simulink model "rwa_power_model_test"  (R2018b)
settings: Solver=VariableStepAuto  StartTime=0.0  StopTime=10.0  RelTol=1e-3
undefined symbols (not defined in the file): simParams
libraries: rwa_power_lib x1, rwa_zero_torque_power_lib x1
settings Model: Creator=Taylor  LastModifiedBy=Taylor

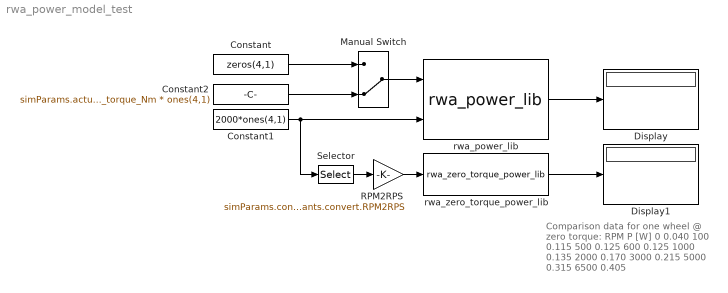
== system rwa_power_model_test ==
  note: Comparison data for one wheel
      | @ zero torque:
      |
      | RPM
      | P [W]
      |
      | 0
      | 0.040
      |
      | 100
      | 0.115
      |
      | 500
      | 0.125
      |
      | 600
      | 0.125
      |
      | 1000
      | 0.135
      |
      | 2000
      | 0.170
      |
      | 3000
      | 0.215
      |
      | 5000
      | 0.315
      |
      | 6500
      | 0.405
  Constant : Constant  Value=zeros(4,1)
  Constant1 : Constant  Value=2000*ones(4,1)
  Constant2 : Constant  Value=simParams.actuators.rwa.max_torque_Nm * ones(4,1)
  Display : Display
  Display1 : Display
  Manual Switch : ManualSwitch  CurrentSetting=0
  RPM2RPS : Gain  Gain=simParams.constants.convert.RPM2RPS
  Selector : Selector  InputPortWidth=4  IndexOptions=Index vector (dialog)  Indices=1  OutputSizes=1
  rwa_power_lib : rwa_power_lib/rwa_power_lib  SystemSampleTime=-1
  rwa_zero_torque_power_lib : rwa_zero_torque_power_lib/rwa_zero_torque_power_lib  SystemSampleTime=-1
  wires:
  Constant/1 -> Manual Switch/1
  Constant1/1 -> rwa_power_lib/2, Selector/1
  rwa_power_lib/1 -> Display/1
  Selector/1 -> RPM2RPS/1
  rwa_zero_torque_power_lib/1 -> Display1/1
  RPM2RPS/1 -> rwa_zero_torque_power_lib/1
  Manual Switch/1 -> rwa_power_lib/1
  Constant2/1 -> Manual Switch/2
